simulink model "FSAC2021"  (R2014a)
settings: Solver=FixedStepDiscrete  StartTime=0.0  StopTime=inf  FixedStep=0.0005  RelTol=1e-3
model workspace (MAT data in the model file):
  MCOS : class17 (value not decoded)
  MCOS : class17 (value not decoded)
  MCOS : class17 (value not decoded)
  MCOS : class17 (value not decoded)
  MCOS : class17 (value not decoded)
  MCOS : class17 (value not decoded)
  MCOS : class17 (value not decoded)
  MCOS : class17 (value not decoded)
  MCOS : class17 (value not decoded)
  MCOS : class17 (value not decoded)
  MCOS : class17 (value not decoded)
  MCOS : class17 (value not decoded)
  MCOS : class17 (value not decoded)
  MCOS : class17 (value not decoded)
  MCOS : class17 (value not decoded)
  MCOS : class17 (value not decoded)
  MCOS : class17 (value not decoded)
  MCOS : class17 (value not decoded)
  MCOS : class17 (value not decoded)
  BUZZER_START = 1
  MCOS : class17 (value not decoded)
  MCOS : class17 (value not decoded)
  MCOS : class17 (value not decoded)
  MCOS : class17 (value not decoded)
  MCOS : class17 (value not decoded)
  MCOS : class17 (value not decoded)
  MCOS : class17 (value not decoded)
  MCOS : class17 (value not decoded)
  MCOS : class17 (value not decoded)
  MCOS : class17 (value not decoded)
  MCOS : class17 (value not decoded)
  MCOS : class17 (value not decoded)
  MCOS : class17 (value not decoded)
  MCOS : class17 (value not decoded)
  MCOS : class17 (value not decoded)
  MCOS : class17 (value not decoded)
  MCOS : class17 (value not decoded)
  MCOS : class17 (value not decoded)
  MCOS : class17 (value not decoded)
  MCOS : class17 (value not decoded)
  MCOS : class17 (value not decoded)
  MCOS : class17 (value not decoded)
  MCOS : class17 (value not decoded)
  MCOS : class17 (value not decoded)
  MCOS : class17 (value not decoded)
  MCOS : class17 (value not decoded)
  MCOS : class17 (value not decoded)
  MCOS : class17 (value not decoded)
  MCOS : class17 (value not decoded)
  MCOS : class17 (value not decoded)
  MCOS : class17 (value not decoded)
  MCOS : class17 (value not decoded)
  MCOS : class17 (value not decoded)
  MCOS : class17 (value not decoded)
  MCOS : class17 (value not decoded)
  MCOS : class17 (value not decoded)
  MCOS : class17 (value not decoded)
  MCOS : class17 (value not decoded)
  Brake = 11
  MCOS : class17 (value not decoded)
  MCOS : class17 (value not decoded)
  MCOS : class17 (value not decoded)
  MCOS : class17 (value not decoded)
  MCOS : class17 (value not decoded)
  MCOS : class17 (value not decoded)
  MCOS : class17 (value not decoded)
  MCOS : class17 (value not decoded)
  Sensor_Acc_b = 101.85
  Sensor_Acc_k = -0.0185
  Str_Sen_Orig_Angle = -341
  MCOS : class17 (value not decoded)
  Tire_D = 0.47
  T = 0.05
libraries: simulink x396, ec55xxlib x126
(part 17 of 17)

== system FSAC2021/ROUTING/TO_DCAN/Subsystem/DIAG_VEH_SENSOR/Front_wheel_angle ==
  Front_wheel_angle : Inport
  Constant{1..3,5..8} (7 alike) : Constant  Value=0  OutDataTypeStr=uint8  SampleTime=-1
  Front_wheel_angleABS : Abs
  Front_wheel_angleCS : ArithShift  BitShiftNumber=-8
  Front_wheel_angleConS : Constant  OutDataTypeStr=single
  Front_wheel_angleCosR : Constant  Value=0  OutDataTypeStr=uint8
  Front_wheel_angleROP : RelationalOperator  Operator=<  OutDataTypeStr=boolean
  Front_wheel_angleRon : Rounding  Operator=round
  Front_wheel_angleSW : Switch  Criteria=u2 ~= 0
  Front_wheel_angle_1sat : Saturate  UpperLimit=255  LowerLimit=0
  Front_wheel_angle_Convert : DataTypeConversion  OutDataTypeStr=uint8
  Front_wheel_angle_Convert1 : DataTypeConversion  OutDataTypeStr=uint32
  Front_wheel_angle_D : Product  Inputs=*/
  Front_wheel_angle_F : Constant  OutDataTypeStr=single
  Front_wheel_angle_L : simulink/Logic and Bit Operations/Bitwise Operator  logicop=AND  UseBitMask=on  BitMask=255  BitMaskRealWorld=Stored Integer
  Front_wheel_angle_O : Constant  Value=0  OutDataTypeStr=single
  Front_wheel_angle_S : ArithShift
  Front_wheel_angle_sat : Saturate  UpperLimit=127  LowerLimit=-128
  Front_wheel_angle_st : Sum  Inputs=+-
  Front_wheel_anglesubcon : Sum  Inputs=+-
  output1 : Outport
  output2 : Outport  Port=2
  output3 : Outport  Port=3
  output4 : Outport  Port=4
  output5 : Outport  Port=5
  output6 : Outport  Port=6
  output7 : Outport  Port=7
  output8 : Outport  Port=8
  wires:
  Front_wheel_angle/1 -> Front_wheel_angle_sat/1
  Front_wheel_angle_sat/1 -> Front_wheel_angle_st/1
  Front_wheel_angle_O/1 -> Front_wheel_angle_st/2
  Front_wheel_angle_st/1 -> Front_wheel_angle_D/1
  Front_wheel_angle_F/1 -> Front_wheel_angle_D/2
  Front_wheel_angle_D/1 -> Front_wheel_angleRon/1
  Front_wheel_angleRon/1 -> Front_wheel_angleROP/1, Front_wheel_angleABS/1, Front_wheel_angleSW/3
  Front_wheel_angleCosR/1 -> Front_wheel_angleROP/2
  Front_wheel_angleConS/1 -> Front_wheel_angleCS/1
  Front_wheel_angleCS/1 -> Front_wheel_anglesubcon/1
  Front_wheel_angleABS/1 -> Front_wheel_anglesubcon/2
  Front_wheel_anglesubcon/1 -> Front_wheel_angleSW/1
  Front_wheel_angleROP/1 -> Front_wheel_angleSW/2
  Front_wheel_angleSW/1 -> Front_wheel_angle_S/1
  Front_wheel_angle_S/1 -> Front_wheel_angle_1sat/1
  Front_wheel_angle_1sat/1 -> Front_wheel_angle_Convert1/1
  Front_wheel_angle_Convert1/1 -> Front_wheel_angle_L/1
  Front_wheel_angle_L/1 -> Front_wheel_angle_Convert/1
  Front_wheel_angle_Convert/1 -> output4/1
  Constant1/1 -> output1/1
  Constant2/1 -> output2/1
  Constant3/1 -> output3/1
  Constant5/1 -> output5/1
  Constant6/1 -> output6/1
  Constant7/1 -> output7/1
  Constant8/1 -> output8/1

== system FSAC2021/ROUTING/TO_DCAN/Subsystem/DIAG_VEH_SENSOR/Hydra_Prs ==
  Hydra_Prs : Inport
  Constant{1..4,6..8} (7 alike) : Constant  Value=0  OutDataTypeStr=uint8  SampleTime=-1
  Hydra_PrsRon : Rounding  Operator=round
  Hydra_Prs_1sat : Saturate  UpperLimit=255  LowerLimit=0
  Hydra_Prs_Convert : DataTypeConversion  OutDataTypeStr=uint8
  Hydra_Prs_Convert1 : DataTypeConversion  OutDataTypeStr=uint32
  Hydra_Prs_D : Product  Inputs=*/
  Hydra_Prs_F : Constant  Value=0.1  OutDataTypeStr=single
  Hydra_Prs_L : simulink/Logic and Bit Operations/Bitwise Operator  logicop=AND  UseBitMask=on  BitMask=255  BitMaskRealWorld=Stored Integer
  Hydra_Prs_O : Constant  Value=0  OutDataTypeStr=single
  Hydra_Prs_S : ArithShift
  Hydra_Prs_sat : Saturate  UpperLimit=25.5  LowerLimit=0
  Hydra_Prs_st : Sum  Inputs=+-
  output1 : Outport
  output2 : Outport  Port=2
  output3 : Outport  Port=3
  output4 : Outport  Port=4
  output5 : Outport  Port=5
  output6 : Outport  Port=6
  output7 : Outport  Port=7
  output8 : Outport  Port=8
  wires:
  Hydra_Prs/1 -> Hydra_Prs_sat/1
  Hydra_Prs_sat/1 -> Hydra_Prs_st/1
  Hydra_Prs_O/1 -> Hydra_Prs_st/2
  Hydra_Prs_st/1 -> Hydra_Prs_D/1
  Hydra_Prs_F/1 -> Hydra_Prs_D/2
  Hydra_Prs_D/1 -> Hydra_PrsRon/1
  Hydra_PrsRon/1 -> Hydra_Prs_S/1
  Hydra_Prs_S/1 -> Hydra_Prs_1sat/1
  Hydra_Prs_1sat/1 -> Hydra_Prs_Convert1/1
  Hydra_Prs_Convert1/1 -> Hydra_Prs_L/1
  Hydra_Prs_L/1 -> Hydra_Prs_Convert/1
  Hydra_Prs_Convert/1 -> output5/1
  Constant1/1 -> output1/1
  Constant2/1 -> output2/1
  Constant3/1 -> output3/1
  Constant4/1 -> output4/1
  Constant6/1 -> output6/1
  Constant7/1 -> output7/1
  Constant8/1 -> output8/1

== system FSAC2021/ROUTING/TO_DCAN/Subsystem/DIAG_VEH_SENSOR/Mtr_Input_Volt ==
  Mtr_Input_Volt : Inport
  Constant{1,3..8} (7 alike) : Constant  Value=0  OutDataTypeStr=uint8  SampleTime=-1
  Mtr_Input_VoltRon : Rounding  Operator=round
  Mtr_Input_Volt_1sat : Saturate  UpperLimit=255  LowerLimit=0
  Mtr_Input_Volt_Convert : DataTypeConversion  OutDataTypeStr=uint8
  Mtr_Input_Volt_Convert1 : DataTypeConversion  OutDataTypeStr=uint32
  Mtr_Input_Volt_D : Product  Inputs=*/
  Mtr_Input_Volt_F : Constant  OutDataTypeStr=single
  Mtr_Input_Volt_L : simulink/Logic and Bit Operations/Bitwise Operator  logicop=AND  UseBitMask=on  BitMask=255  BitMaskRealWorld=Stored Integer
  Mtr_Input_Volt_O : Constant  Value=0  OutDataTypeStr=single
  Mtr_Input_Volt_S : ArithShift
  Mtr_Input_Volt_sat : Saturate  UpperLimit=255  LowerLimit=0
  Mtr_Input_Volt_st : Sum  Inputs=+-
  output1 : Outport
  output2 : Outport  Port=2
  output3 : Outport  Port=3
  output4 : Outport  Port=4
  output5 : Outport  Port=5
  output6 : Outport  Port=6
  output7 : Outport  Port=7
  output8 : Outport  Port=8
  wires:
  Mtr_Input_Volt/1 -> Mtr_Input_Volt_sat/1
  Mtr_Input_Volt_sat/1 -> Mtr_Input_Volt_st/1
  Mtr_Input_Volt_O/1 -> Mtr_Input_Volt_st/2
  Mtr_Input_Volt_st/1 -> Mtr_Input_Volt_D/1
  Mtr_Input_Volt_F/1 -> Mtr_Input_Volt_D/2
  Mtr_Input_Volt_D/1 -> Mtr_Input_VoltRon/1
  Mtr_Input_VoltRon/1 -> Mtr_Input_Volt_S/1
  Mtr_Input_Volt_S/1 -> Mtr_Input_Volt_1sat/1
  Mtr_Input_Volt_1sat/1 -> Mtr_Input_Volt_Convert1/1
  Mtr_Input_Volt_Convert1/1 -> Mtr_Input_Volt_L/1
  Mtr_Input_Volt_L/1 -> Mtr_Input_Volt_Convert/1
  Mtr_Input_Volt_Convert/1 -> output2/1
  Constant1/1 -> output1/1
  Constant3/1 -> output3/1
  Constant4/1 -> output4/1
  Constant5/1 -> output5/1
  Constant6/1 -> output6/1
  Constant7/1 -> output7/1
  Constant8/1 -> output8/1

== system FSAC2021/ROUTING/TO_DCAN/Subsystem/DIAG_VEH_SENSOR/Pedal_Acc ==
  Pedal_Acc : Inport
  Constant{1..6} (6 alike) : Constant  Value=0  OutDataTypeStr=uint8  SampleTime=-1
  Pedal_AccBitCov : DataTypeConversion  OutDataTypeStr=uint8
  Pedal_AccCOV : DataTypeConversion  OutDataTypeStr=uint8
  Pedal_AccRon : Rounding  Operator=round
  Pedal_Acc_1sat : Saturate  UpperLimit=16256  LowerLimit=0
  Pedal_Acc_And : simulink/Logic and Bit Operations/Bitwise Operator  logicop=AND  UseBitMask=off  NumInputPorts=2  BitMask=bin2dec('11011001')  BitMaskRealWorld=Stored Integer
  Pedal_Acc_And_C : Constant  Value=255  OutDataTypeStr=uint32
  Pedal_Acc_Convert : DataTypeConversion  OutDataTypeStr=uint32
  Pedal_Acc_D : Product  Inputs=*/
  Pedal_Acc_D1 : Product  Inputs=*/
  Pedal_Acc_F : Constant  OutDataTypeStr=single
  Pedal_Acc_L : simulink/Logic and Bit Operations/Bitwise Operator  logicop=AND  UseBitMask=on  BitMask=16256  BitMaskRealWorld=Stored Integer
  Pedal_Acc_O : Constant  Value=0  OutDataTypeStr=single
  Pedal_Acc_S : ArithShift  BitShiftNumber=-7
  Pedal_Acc_sat : Saturate  UpperLimit=127  LowerLimit=0
  Pedal_Acc_st : Sum  Inputs=+-
  Pedal_Accoutput7_C : Constant  Value=256
  output1 : Outport
  output2 : Outport  Port=2
  output3 : Outport  Port=3
  output4 : Outport  Port=4
  output5 : Outport  Port=5
  output6 : Outport  Port=6
  output7 : Outport  Port=7
  output8 : Outport  Port=8
  wires:
  Pedal_Acc/1 -> Pedal_Acc_sat/1
  Pedal_Acc_sat/1 -> Pedal_Acc_st/1
  Pedal_Acc_O/1 -> Pedal_Acc_st/2
  Pedal_Acc_st/1 -> Pedal_Acc_D/1
  Pedal_Acc_F/1 -> Pedal_Acc_D/2
  Pedal_Acc_D/1 -> Pedal_AccRon/1
  Pedal_AccRon/1 -> Pedal_Acc_S/1
  Pedal_Acc_S/1 -> Pedal_Acc_1sat/1
  Pedal_Acc_1sat/1 -> Pedal_Acc_Convert/1
  Pedal_Acc_Convert/1 -> Pedal_Acc_L/1
  Pedal_Acc_L/1 -> Pedal_Acc_D1/1, Pedal_Acc_And/1
  Pedal_Accoutput7_C/1 -> Pedal_Acc_D1/2
  Pedal_Acc_D1/1 -> Pedal_AccCOV/1
  Pedal_AccCOV/1 -> output7/1
  Pedal_Acc_And_C/1 -> Pedal_Acc_And/2
  Pedal_Acc_And/1 -> Pedal_AccBitCov/1
  Pedal_AccBitCov/1 -> output8/1
  Constant1/1 -> output1/1
  Constant2/1 -> output2/1
  Constant3/1 -> output3/1
  Constant4/1 -> output4/1
  Constant5/1 -> output5/1
  Constant6/1 -> output6/1

== system FSAC2021/ROUTING/TO_DCAN/Subsystem/DIAG_VEH_SENSOR/Pedal_Brake ==
  Pedal_Brake : Inport
  Constant{1..7} (7 alike) : Constant  Value=0  OutDataTypeStr=uint8  SampleTime=-1
  Pedal_BrakeRon : Rounding  Operator=round
  Pedal_Brake_1sat : Saturate  UpperLimit=127  LowerLimit=0
  Pedal_Brake_Convert : DataTypeConversion  OutDataTypeStr=uint8
  Pedal_Brake_Convert1 : DataTypeConversion  OutDataTypeStr=uint32
  Pedal_Brake_D : Product  Inputs=*/
  Pedal_Brake_F : Constant  OutDataTypeStr=single
  Pedal_Brake_L : simulink/Logic and Bit Operations/Bitwise Operator  logicop=AND  UseBitMask=on  BitMask=127  BitMaskRealWorld=Stored Integer
  Pedal_Brake_O : Constant  Value=0  OutDataTypeStr=single
  Pedal_Brake_S : ArithShift
  Pedal_Brake_sat : Saturate  UpperLimit=127  LowerLimit=0
  Pedal_Brake_st : Sum  Inputs=+-
  output1 : Outport
  output2 : Outport  Port=2
  output3 : Outport  Port=3
  output4 : Outport  Port=4
  output5 : Outport  Port=5
  output6 : Outport  Port=6
  output7 : Outport  Port=7
  output8 : Outport  Port=8
  wires:
  Pedal_Brake/1 -> Pedal_Brake_sat/1
  Pedal_Brake_sat/1 -> Pedal_Brake_st/1
  Pedal_Brake_O/1 -> Pedal_Brake_st/2
  Pedal_Brake_st/1 -> Pedal_Brake_D/1
  Pedal_Brake_F/1 -> Pedal_Brake_D/2
  Pedal_Brake_D/1 -> Pedal_BrakeRon/1
  Pedal_BrakeRon/1 -> Pedal_Brake_S/1
  Pedal_Brake_S/1 -> Pedal_Brake_1sat/1
  Pedal_Brake_1sat/1 -> Pedal_Brake_Convert1/1
  Pedal_Brake_Convert1/1 -> Pedal_Brake_L/1
  Pedal_Brake_L/1 -> Pedal_Brake_Convert/1
  Pedal_Brake_Convert/1 -> output8/1
  Constant1/1 -> output1/1
  Constant2/1 -> output2/1
  Constant3/1 -> output3/1
  Constant4/1 -> output4/1
  Constant5/1 -> output5/1
  Constant6/1 -> output6/1
  Constant7/1 -> output7/1

== system FSAC2021/ROUTING/TO_DCAN/Subsystem/DIAG_VEH_SENSOR/Veh_Current_Speed ==
  Veh_Current_Speed : Inport
  Constant{1..5,8} (6 alike) : Constant  Value=0  OutDataTypeStr=uint8  SampleTime=-1
  Veh_Current_SpeedBitCov : DataTypeConversion  OutDataTypeStr=uint8
  Veh_Current_SpeedCOV : DataTypeConversion  OutDataTypeStr=uint8
  Veh_Current_SpeedRon : Rounding  Operator=round
  Veh_Current_Speed_1sat : Saturate  UpperLimit=65472  LowerLimit=0
  Veh_Current_Speed_And : simulink/Logic and Bit Operations/Bitwise Operator  logicop=AND  UseBitMask=off  NumInputPorts=2  BitMask=bin2dec('11011001')  BitMaskRealWorld=Stored Integer
  Veh_Current_Speed_And_C : Constant  Value=255  OutDataTypeStr=uint32
  Veh_Current_Speed_Convert : DataTypeConversion  OutDataTypeStr=uint32
  Veh_Current_Speed_D : Product  Inputs=*/
  Veh_Current_Speed_D1 : Product  Inputs=*/
  Veh_Current_Speed_F : Constant  Value=0.1  OutDataTypeStr=single
  Veh_Current_Speed_L : simulink/Logic and Bit Operations/Bitwise Operator  logicop=AND  UseBitMask=on  BitMask=65472  BitMaskRealWorld=Stored Integer
  Veh_Current_Speed_O : Constant  Value=0  OutDataTypeStr=single
  Veh_Current_Speed_S : ArithShift  BitShiftNumber=-6
  Veh_Current_Speed_sat : Saturate  UpperLimit=102.3  LowerLimit=0
  Veh_Current_Speed_st : Sum  Inputs=+-
  Veh_Current_Speedoutput6_C : Constant  Value=256
  output1 : Outport
  output2 : Outport  Port=2
  output3 : Outport  Port=3
  output4 : Outport  Port=4
  output5 : Outport  Port=5
  output6 : Outport  Port=6
  output7 : Outport  Port=7
  output8 : Outport  Port=8
  wires:
  Veh_Current_Speed/1 -> Veh_Current_Speed_sat/1
  Veh_Current_Speed_sat/1 -> Veh_Current_Speed_st/1
  Veh_Current_Speed_O/1 -> Veh_Current_Speed_st/2
  Veh_Current_Speed_st/1 -> Veh_Current_Speed_D/1
  Veh_Current_Speed_F/1 -> Veh_Current_Speed_D/2
  Veh_Current_Speed_D/1 -> Veh_Current_SpeedRon/1
  Veh_Current_SpeedRon/1 -> Veh_Current_Speed_S/1
  Veh_Current_Speed_S/1 -> Veh_Current_Speed_1sat/1
  Veh_Current_Speed_1sat/1 -> Veh_Current_Speed_Convert/1
  Veh_Current_Speed_Convert/1 -> Veh_Current_Speed_L/1
  Veh_Current_Speed_L/1 -> Veh_Current_Speed_D1/1, Veh_Current_Speed_And/1
  Veh_Current_Speedoutput6_C/1 -> Veh_Current_Speed_D1/2
  Veh_Current_Speed_D1/1 -> Veh_Current_SpeedCOV/1
  Veh_Current_SpeedCOV/1 -> output6/1
  Veh_Current_Speed_And_C/1 -> Veh_Current_Speed_And/2
  Veh_Current_Speed_And/1 -> Veh_Current_SpeedBitCov/1
  Veh_Current_SpeedBitCov/1 -> output7/1
  Constant1/1 -> output1/1
  Constant2/1 -> output2/1
  Constant3/1 -> output3/1
  Constant4/1 -> output4/1
  Constant5/1 -> output5/1
  Constant8/1 -> output8/1

== system FSAC2021/ROUTING/TO_DCAN/Subsystem/DIAG_WHL_SPD/FL_Whl_Spd ==
  FL_Whl_Spd : Inport
  Constant{3..8} (6 alike) : Constant  Value=0  OutDataTypeStr=uint8  SampleTime=-1
  FL_Whl_SpdBitCov : DataTypeConversion  OutDataTypeStr=uint8
  FL_Whl_SpdCOV : DataTypeConversion  OutDataTypeStr=uint8
  FL_Whl_SpdRon : Rounding  Operator=round
  FL_Whl_Spd_1sat : Saturate  UpperLimit=65535  LowerLimit=0
  FL_Whl_Spd_And : simulink/Logic and Bit Operations/Bitwise Operator  logicop=AND  UseBitMask=off  NumInputPorts=2  BitMask=bin2dec('11011001')  BitMaskRealWorld=Stored Integer
  FL_Whl_Spd_And_C : Constant  Value=255  OutDataTypeStr=uint32
  FL_Whl_Spd_Convert : DataTypeConversion  OutDataTypeStr=uint32
  FL_Whl_Spd_D : Product  Inputs=*/
  FL_Whl_Spd_D1 : Product  Inputs=*/
  FL_Whl_Spd_F : Constant  OutDataTypeStr=single
  FL_Whl_Spd_L : simulink/Logic and Bit Operations/Bitwise Operator  logicop=AND  UseBitMask=on  BitMask=65535  BitMaskRealWorld=Stored Integer
  FL_Whl_Spd_O : Constant  Value=0  OutDataTypeStr=single
  FL_Whl_Spd_S : ArithShift
  FL_Whl_Spd_sat : Saturate  UpperLimit=65535  LowerLimit=0
  FL_Whl_Spd_st : Sum  Inputs=+-
  FL_Whl_Spdoutput1_C : Constant  Value=256
  output1 : Outport
  output2 : Outport  Port=2
  output3 : Outport  Port=3
  output4 : Outport  Port=4
  output5 : Outport  Port=5
  output6 : Outport  Port=6
  output7 : Outport  Port=7
  output8 : Outport  Port=8
  wires:
  FL_Whl_Spd/1 -> FL_Whl_Spd_sat/1
  FL_Whl_Spd_sat/1 -> FL_Whl_Spd_st/1
  FL_Whl_Spd_O/1 -> FL_Whl_Spd_st/2
  FL_Whl_Spd_st/1 -> FL_Whl_Spd_D/1
  FL_Whl_Spd_F/1 -> FL_Whl_Spd_D/2
  FL_Whl_Spd_D/1 -> FL_Whl_SpdRon/1
  FL_Whl_SpdRon/1 -> FL_Whl_Spd_S/1
  FL_Whl_Spd_S/1 -> FL_Whl_Spd_1sat/1
  FL_Whl_Spd_1sat/1 -> FL_Whl_Spd_Convert/1
  FL_Whl_Spd_Convert/1 -> FL_Whl_Spd_L/1
  FL_Whl_Spd_L/1 -> FL_Whl_Spd_D1/1, FL_Whl_Spd_And/1
  FL_Whl_Spdoutput1_C/1 -> FL_Whl_Spd_D1/2
  FL_Whl_Spd_D1/1 -> FL_Whl_SpdCOV/1
  FL_Whl_SpdCOV/1 -> output1/1
  FL_Whl_Spd_And_C/1 -> FL_Whl_Spd_And/2
  FL_Whl_Spd_And/1 -> FL_Whl_SpdBitCov/1
  FL_Whl_SpdBitCov/1 -> output2/1
  Constant3/1 -> output3/1
  Constant4/1 -> output4/1
  Constant5/1 -> output5/1
  Constant6/1 -> output6/1
  Constant7/1 -> output7/1
  Constant8/1 -> output8/1

== system FSAC2021/ROUTING/TO_DCAN/Subsystem/DIAG_WHL_SPD/FR_Whl_Spd ==
  FR_Whl_Spd : Inport
  Constant{1..2,5..8} (6 alike) : Constant  Value=0  OutDataTypeStr=uint8  SampleTime=-1
  FR_Whl_SpdBitCov : DataTypeConversion  OutDataTypeStr=uint8
  FR_Whl_SpdCOV : DataTypeConversion  OutDataTypeStr=uint8
  FR_Whl_SpdRon : Rounding  Operator=round
  FR_Whl_Spd_1sat : Saturate  UpperLimit=65535  LowerLimit=0
  FR_Whl_Spd_And : simulink/Logic and Bit Operations/Bitwise Operator  logicop=AND  UseBitMask=off  NumInputPorts=2  BitMask=bin2dec('11011001')  BitMaskRealWorld=Stored Integer
  FR_Whl_Spd_And_C : Constant  Value=255  OutDataTypeStr=uint32
  FR_Whl_Spd_Convert : DataTypeConversion  OutDataTypeStr=uint32
  FR_Whl_Spd_D : Product  Inputs=*/
  FR_Whl_Spd_D1 : Product  Inputs=*/
  FR_Whl_Spd_F : Constant  OutDataTypeStr=single
  FR_Whl_Spd_L : simulink/Logic and Bit Operations/Bitwise Operator  logicop=AND  UseBitMask=on  BitMask=65535  BitMaskRealWorld=Stored Integer
  FR_Whl_Spd_O : Constant  Value=0  OutDataTypeStr=single
  FR_Whl_Spd_S : ArithShift
  FR_Whl_Spd_sat : Saturate  UpperLimit=65535  LowerLimit=0
  FR_Whl_Spd_st : Sum  Inputs=+-
  FR_Whl_Spdoutput3_C : Constant  Value=256
  output1 : Outport
  output2 : Outport  Port=2
  output3 : Outport  Port=3
  output4 : Outport  Port=4
  output5 : Outport  Port=5
  output6 : Outport  Port=6
  output7 : Outport  Port=7
  output8 : Outport  Port=8
  wires:
  FR_Whl_Spd/1 -> FR_Whl_Spd_sat/1
  FR_Whl_Spd_sat/1 -> FR_Whl_Spd_st/1
  FR_Whl_Spd_O/1 -> FR_Whl_Spd_st/2
  FR_Whl_Spd_st/1 -> FR_Whl_Spd_D/1
  FR_Whl_Spd_F/1 -> FR_Whl_Spd_D/2
  FR_Whl_Spd_D/1 -> FR_Whl_SpdRon/1
  FR_Whl_SpdRon/1 -> FR_Whl_Spd_S/1
  FR_Whl_Spd_S/1 -> FR_Whl_Spd_1sat/1
  FR_Whl_Spd_1sat/1 -> FR_Whl_Spd_Convert/1
  FR_Whl_Spd_Convert/1 -> FR_Whl_Spd_L/1
  FR_Whl_Spd_L/1 -> FR_Whl_Spd_D1/1, FR_Whl_Spd_And/1
  FR_Whl_Spdoutput3_C/1 -> FR_Whl_Spd_D1/2
  FR_Whl_Spd_D1/1 -> FR_Whl_SpdCOV/1
  FR_Whl_SpdCOV/1 -> output3/1
  FR_Whl_Spd_And_C/1 -> FR_Whl_Spd_And/2
  FR_Whl_Spd_And/1 -> FR_Whl_SpdBitCov/1
  FR_Whl_SpdBitCov/1 -> output4/1
  Constant1/1 -> output1/1
  Constant2/1 -> output2/1
  Constant5/1 -> output5/1
  Constant6/1 -> output6/1
  Constant7/1 -> output7/1
  Constant8/1 -> output8/1

== system FSAC2021/ROUTING/TO_DCAN/Subsystem/DIAG_WHL_SPD/RL_Whl_Spd ==
  RL_Whl_Spd : Inport
  Constant{1..4,7..8} (6 alike) : Constant  Value=0  OutDataTypeStr=uint8  SampleTime=-1
  RL_Whl_SpdBitCov : DataTypeConversion  OutDataTypeStr=uint8
  RL_Whl_SpdCOV : DataTypeConversion  OutDataTypeStr=uint8
  RL_Whl_SpdRon : Rounding  Operator=round
  RL_Whl_Spd_1sat : Saturate  UpperLimit=65535  LowerLimit=0
  RL_Whl_Spd_And : simulink/Logic and Bit Operations/Bitwise Operator  logicop=AND  UseBitMask=off  NumInputPorts=2  BitMask=bin2dec('11011001')  BitMaskRealWorld=Stored Integer
  RL_Whl_Spd_And_C : Constant  Value=255  OutDataTypeStr=uint32
  RL_Whl_Spd_Convert : DataTypeConversion  OutDataTypeStr=uint32
  RL_Whl_Spd_D : Product  Inputs=*/
  RL_Whl_Spd_D1 : Product  Inputs=*/
  RL_Whl_Spd_F : Constant  OutDataTypeStr=single
  RL_Whl_Spd_L : simulink/Logic and Bit Operations/Bitwise Operator  logicop=AND  UseBitMask=on  BitMask=65535  BitMaskRealWorld=Stored Integer
  RL_Whl_Spd_O : Constant  Value=0  OutDataTypeStr=single
  RL_Whl_Spd_S : ArithShift
  RL_Whl_Spd_sat : Saturate  UpperLimit=65535  LowerLimit=0
  RL_Whl_Spd_st : Sum  Inputs=+-
  RL_Whl_Spdoutput5_C : Constant  Value=256
  output1 : Outport
  output2 : Outport  Port=2
  output3 : Outport  Port=3
  output4 : Outport  Port=4
  output5 : Outport  Port=5
  output6 : Outport  Port=6
  output7 : Outport  Port=7
  output8 : Outport  Port=8
  wires:
  RL_Whl_Spd/1 -> RL_Whl_Spd_sat/1
  RL_Whl_Spd_sat/1 -> RL_Whl_Spd_st/1
  RL_Whl_Spd_O/1 -> RL_Whl_Spd_st/2
  RL_Whl_Spd_st/1 -> RL_Whl_Spd_D/1
  RL_Whl_Spd_F/1 -> RL_Whl_Spd_D/2
  RL_Whl_Spd_D/1 -> RL_Whl_SpdRon/1
  RL_Whl_SpdRon/1 -> RL_Whl_Spd_S/1
  RL_Whl_Spd_S/1 -> RL_Whl_Spd_1sat/1
  RL_Whl_Spd_1sat/1 -> RL_Whl_Spd_Convert/1
  RL_Whl_Spd_Convert/1 -> RL_Whl_Spd_L/1
  RL_Whl_Spd_L/1 -> RL_Whl_Spd_D1/1, RL_Whl_Spd_And/1
  RL_Whl_Spdoutput5_C/1 -> RL_Whl_Spd_D1/2
  RL_Whl_Spd_D1/1 -> RL_Whl_SpdCOV/1
  RL_Whl_SpdCOV/1 -> output5/1
  RL_Whl_Spd_And_C/1 -> RL_Whl_Spd_And/2
  RL_Whl_Spd_And/1 -> RL_Whl_SpdBitCov/1
  RL_Whl_SpdBitCov/1 -> output6/1
  Constant1/1 -> output1/1
  Constant2/1 -> output2/1
  Constant3/1 -> output3/1
  Constant4/1 -> output4/1
  Constant7/1 -> output7/1
  Constant8/1 -> output8/1

== system FSAC2021/ROUTING/TO_DCAN/Subsystem/DIAG_WHL_SPD/RR_Whl_Spd ==
  RR_Whl_Spd : Inport
  Constant{1..6} (6 alike) : Constant  Value=0  OutDataTypeStr=uint8  SampleTime=-1
  RR_Whl_SpdBitCov : DataTypeConversion  OutDataTypeStr=uint8
  RR_Whl_SpdCOV : DataTypeConversion  OutDataTypeStr=uint8
  RR_Whl_SpdRon : Rounding  Operator=round
  RR_Whl_Spd_1sat : Saturate  UpperLimit=65535  LowerLimit=0
  RR_Whl_Spd_And : simulink/Logic and Bit Operations/Bitwise Operator  logicop=AND  UseBitMask=off  NumInputPorts=2  BitMask=bin2dec('11011001')  BitMaskRealWorld=Stored Integer
  RR_Whl_Spd_And_C : Constant  Value=255  OutDataTypeStr=uint32
  RR_Whl_Spd_Convert : DataTypeConversion  OutDataTypeStr=uint32
  RR_Whl_Spd_D : Product  Inputs=*/
  RR_Whl_Spd_D1 : Product  Inputs=*/
  RR_Whl_Spd_F : Constant  OutDataTypeStr=single
  RR_Whl_Spd_L : simulink/Logic and Bit Operations/Bitwise Operator  logicop=AND  UseBitMask=on  BitMask=65535  BitMaskRealWorld=Stored Integer
  RR_Whl_Spd_O : Constant  Value=0  OutDataTypeStr=single
  RR_Whl_Spd_S : ArithShift
  RR_Whl_Spd_sat : Saturate  UpperLimit=65535  LowerLimit=0
  RR_Whl_Spd_st : Sum  Inputs=+-
  RR_Whl_Spdoutput7_C : Constant  Value=256
  output1 : Outport
  output2 : Outport  Port=2
  output3 : Outport  Port=3
  output4 : Outport  Port=4
  output5 : Outport  Port=5
  output6 : Outport  Port=6
  output7 : Outport  Port=7
  output8 : Outport  Port=8
  wires:
  RR_Whl_Spd/1 -> RR_Whl_Spd_sat/1
  RR_Whl_Spd_sat/1 -> RR_Whl_Spd_st/1
  RR_Whl_Spd_O/1 -> RR_Whl_Spd_st/2
  RR_Whl_Spd_st/1 -> RR_Whl_Spd_D/1
  RR_Whl_Spd_F/1 -> RR_Whl_Spd_D/2
  RR_Whl_Spd_D/1 -> RR_Whl_SpdRon/1
  RR_Whl_SpdRon/1 -> RR_Whl_Spd_S/1
  RR_Whl_Spd_S/1 -> RR_Whl_Spd_1sat/1
  RR_Whl_Spd_1sat/1 -> RR_Whl_Spd_Convert/1
  RR_Whl_Spd_Convert/1 -> RR_Whl_Spd_L/1
  RR_Whl_Spd_L/1 -> RR_Whl_Spd_D1/1, RR_Whl_Spd_And/1
  RR_Whl_Spdoutput7_C/1 -> RR_Whl_Spd_D1/2
  RR_Whl_Spd_D1/1 -> RR_Whl_SpdCOV/1
  RR_Whl_SpdCOV/1 -> output7/1
  RR_Whl_Spd_And_C/1 -> RR_Whl_Spd_And/2
  RR_Whl_Spd_And/1 -> RR_Whl_SpdBitCov/1
  RR_Whl_SpdBitCov/1 -> output8/1
  Constant1/1 -> output1/1
  Constant2/1 -> output2/1
  Constant3/1 -> output3/1
  Constant4/1 -> output4/1
  Constant5/1 -> output5/1
  Constant6/1 -> output6/1

== system FSAC2021/VCU_CAN_Read/PCANA(RES、AMI、MOTEC、BRAKE、STEER_SENSOR、IPC)/MOTEC_MOTION /MOTEC_MOTION/Motec_Currt_Ang_Sub ==
  In1 : Inport
  Out1 : Outport
  wires:
  In1/1 -> Out1/1

== system FSAC2021/VCU_CAN_Read/PCANA(RES、AMI、MOTEC、BRAKE、STEER_SENSOR、IPC)/MOTEC_MOTION /MOTEC_MOTION/Motec_Currt_Current_Sub ==
  In1 : Inport
  Out1 : Outport
  wires:
  In1/1 -> Out1/1

== system FSAC2021/VCU_CAN_Read/PCANA(RES、AMI、MOTEC、BRAKE、STEER_SENSOR、IPC)/MOTEC_MOTION /MOTEC_MOTION/Motec_Currt_Position_Sub ==
  In1 : Inport
  Out1 : Outport
  wires:
  In1/1 -> Out1/1

== system FSAC2021/VCU_CAN_Read/PCANA(RES、AMI、MOTEC、BRAKE、STEER_SENSOR、IPC)/Str_Emergency /MOTEC_EMERGENCY/Str_Curr_Error_Fault_Sub ==
  In1 : Inport
  Out1 : Outport
  wires:
  In1/1 -> Out1/1

== system FSAC2021/VCU_CAN_Read/PCANA(RES、AMI、MOTEC、BRAKE、STEER_SENSOR、IPC)/Str_Emergency /MOTEC_EMERGENCY/Str_Encoder_Error_Sub ==
  In1 : Inport
  Out1 : Outport
  wires:
  In1/1 -> Out1/1

== system FSAC2021/VCU_CAN_Read/PCANA(RES、AMI、MOTEC、BRAKE、STEER_SENSOR、IPC)/Str_Emergency /MOTEC_EMERGENCY/Str_Flash_Error_Sub ==
  In1 : Inport
  Out1 : Outport
  wires:
  In1/1 -> Out1/1

== system FSAC2021/VCU_CAN_Read/PCANA(RES、AMI、MOTEC、BRAKE、STEER_SENSOR、IPC)/Str_Emergency /MOTEC_EMERGENCY/Str_I2t_Alarm_Sub ==
  In1 : Inport
  Out1 : Outport
  wires:
  In1/1 -> Out1/1

== system FSAC2021/VCU_CAN_Read/PCANA(RES、AMI、MOTEC、BRAKE、STEER_SENSOR、IPC)/Str_Emergency /MOTEC_EMERGENCY/Str_I2t_Warning_Sub ==
  In1 : Inport
  Out1 : Outport
  wires:
  In1/1 -> Out1/1

== system FSAC2021/VCU_CAN_Read/PCANA(RES、AMI、MOTEC、BRAKE、STEER_SENSOR、IPC)/Str_Emergency /MOTEC_EMERGENCY/Str_Limit_Pos_Alarm_Sub ==
  In1 : Inport
  Out1 : Outport
  wires:
  In1/1 -> Out1/1

== system FSAC2021/VCU_CAN_Read/PCANA(RES、AMI、MOTEC、BRAKE、STEER_SENSOR、IPC)/Str_Emergency /MOTEC_EMERGENCY/Str_Over_PosError_Sub ==
  In1 : Inport
  Out1 : Outport
  wires:
  In1/1 -> Out1/1

== system FSAC2021/VCU_CAN_Read/PCANA(RES、AMI、MOTEC、BRAKE、STEER_SENSOR、IPC)/Str_Emergency /MOTEC_EMERGENCY/Str_Over_SpdError_Sub ==
  In1 : Inport
  Out1 : Outport
  wires:
  In1/1 -> Out1/1

== system FSAC2021/VCU_CAN_Read/PCANA(RES、AMI、MOTEC、BRAKE、STEER_SENSOR、IPC)/Str_Emergency /MOTEC_EMERGENCY/Str_Over_TopCurr_Sub ==
  In1 : Inport
  Out1 : Outport
  wires:
  In1/1 -> Out1/1

== system FSAC2021/VCU_CAN_Read/PCANA(RES、AMI、MOTEC、BRAKE、STEER_SENSOR、IPC)/Str_Emergency /MOTEC_EMERGENCY/Str_Overvolt_Warning_Sub ==
  In1 : Inport
  Out1 : Outport
  wires:
  In1/1 -> Out1/1

== system FSAC2021/VCU_CAN_Read/PCANA(RES、AMI、MOTEC、BRAKE、STEER_SENSOR、IPC)/Str_Emergency /MOTEC_EMERGENCY/Str_Para_Error_Sub ==
  In1 : Inport
  Out1 : Outport
  wires:
  In1/1 -> Out1/1

== system FSAC2021/VCU_CAN_Read/PCANA(RES、AMI、MOTEC、BRAKE、STEER_SENSOR、IPC)/Str_Emergency /MOTEC_EMERGENCY/Str_PwrMod_TempHigh_Alarm_Sub ==
  In1 : Inport
  Out1 : Outport
  wires:
  In1/1 -> Out1/1

== system FSAC2021/VCU_CAN_Read/PCANA(RES、AMI、MOTEC、BRAKE、STEER_SENSOR、IPC)/Str_Emergency /MOTEC_EMERGENCY/Str_PwrMod_TempHigh_Warning_Sub ==
  In1 : Inport
  Out1 : Outport
  wires:
  In1/1 -> Out1/1

== system FSAC2021/VCU_CAN_Read/PCANA(RES、AMI、MOTEC、BRAKE、STEER_SENSOR、IPC)/Str_Emergency /MOTEC_EMERGENCY/Str_Spd_Over_Alam_Sub ==
  In1 : Inport
  Out1 : Outport
  wires:
  In1/1 -> Out1/1

== system FSAC2021/VCU_CAN_Read/PCANA(RES、AMI、MOTEC、BRAKE、STEER_SENSOR、IPC)/Str_Emergency /MOTEC_EMERGENCY/Str_System_Error_Sub ==
  In1 : Inport
  Out1 : Outport
  wires:
  In1/1 -> Out1/1

== system FSAC2021/VCU_CAN_Read/PCANA(RES、AMI、MOTEC、BRAKE、STEER_SENSOR、IPC)/Str_Emergency /MOTEC_EMERGENCY/Str_UnderVolt_Warning_Sub ==
  In1 : Inport
  Out1 : Outport
  wires:
  In1/1 -> Out1/1

== system FSAC2021/VCU_CAN_Read/PCANB(BMS、DRIVE_MOTOR)/BMS_ALARM /BMS_HCU_ALARM/ALM_AUX_FAIL_Sub ==
  In1 : Inport
  Out1 : Outport
  wires:
  In1/1 -> Out1/1

== system FSAC2021/VCU_CAN_Read/PCANB(BMS、DRIVE_MOTOR)/BMS_ALARM /BMS_HCU_ALARM/ALM_BATT_DT_Sub ==
  In1 : Inport
  Out1 : Outport
  wires:
  In1/1 -> Out1/1

== system FSAC2021/VCU_CAN_Read/PCANB(BMS、DRIVE_MOTOR)/BMS_ALARM /BMS_HCU_ALARM/ALM_BATT_DV_Sub ==
  In1 : Inport
  Out1 : Outport
  wires:
  In1/1 -> Out1/1

== system FSAC2021/VCU_CAN_Read/PCANB(BMS、DRIVE_MOTOR)/BMS_ALARM /BMS_HCU_ALARM/ALM_BATT_OC_Sub ==
  In1 : Inport
  Out1 : Outport
  wires:
  In1/1 -> Out1/1

== system FSAC2021/VCU_CAN_Read/PCANB(BMS、DRIVE_MOTOR)/BMS_ALARM /BMS_HCU_ALARM/ALM_BATT_OV_Sub ==
  In1 : Inport
  Out1 : Outport
  wires:
  In1/1 -> Out1/1

== system FSAC2021/VCU_CAN_Read/PCANB(BMS、DRIVE_MOTOR)/BMS_ALARM /BMS_HCU_ALARM/ALM_BATT_UC_Sub ==
  In1 : Inport
  Out1 : Outport
  wires:
  In1/1 -> Out1/1

== system FSAC2021/VCU_CAN_Read/PCANB(BMS、DRIVE_MOTOR)/BMS_ALARM /BMS_HCU_ALARM/ALM_BATT_UV_Sub ==
  In1 : Inport
  Out1 : Outport
  wires:
  In1/1 -> Out1/1

== system FSAC2021/VCU_CAN_Read/PCANB(BMS、DRIVE_MOTOR)/BMS_ALARM /BMS_HCU_ALARM/ALM_BMU_FAIL_Sub ==
  In1 : Inport
  Out1 : Outport
  wires:
  In1/1 -> Out1/1

== system FSAC2021/VCU_CAN_Read/PCANB(BMS、DRIVE_MOTOR)/BMS_ALARM /BMS_HCU_ALARM/ALM_BSU_FAULT_Sub ==
  In1 : Inport
  Out1 : Outport
  wires:
  In1/1 -> Out1/1

== system FSAC2021/VCU_CAN_Read/PCANB(BMS、DRIVE_MOTOR)/BMS_ALARM /BMS_HCU_ALARM/ALM_BSU_OFFLINE_Sub ==
  In1 : Inport
  Out1 : Outport
  wires:
  In1/1 -> Out1/1

== system FSAC2021/VCU_CAN_Read/PCANB(BMS、DRIVE_MOTOR)/BMS_ALARM /BMS_HCU_ALARM/ALM_CELL_IBK_Sub ==
  In1 : Inport
  Out1 : Outport
  wires:
  In1/1 -> Out1/1

== system FSAC2021/VCU_CAN_Read/PCANB(BMS、DRIVE_MOTOR)/BMS_ALARM /BMS_HCU_ALARM/ALM_CELL_OT_Sub ==
  In1 : Inport
  Out1 : Outport
  wires:
  In1/1 -> Out1/1

== system FSAC2021/VCU_CAN_Read/PCANB(BMS、DRIVE_MOTOR)/BMS_ALARM /BMS_HCU_ALARM/ALM_CELL_OV_Sub ==
  In1 : Inport
  Out1 : Outport
  wires:
  In1/1 -> Out1/1

== system FSAC2021/VCU_CAN_Read/PCANB(BMS、DRIVE_MOTOR)/BMS_ALARM /BMS_HCU_ALARM/ALM_CELL_TBK_Sub ==
  In1 : Inport
  Out1 : Outport
  wires:
  In1/1 -> Out1/1

== system FSAC2021/VCU_CAN_Read/PCANB(BMS、DRIVE_MOTOR)/BMS_ALARM /BMS_HCU_ALARM/ALM_CELL_UT_Sub ==
  In1 : Inport
  Out1 : Outport
  wires:
  In1/1 -> Out1/1

== system FSAC2021/VCU_CAN_Read/PCANB(BMS、DRIVE_MOTOR)/BMS_ALARM /BMS_HCU_ALARM/ALM_CELL_UV_Sub ==
  In1 : Inport
  Out1 : Outport
  wires:
  In1/1 -> Out1/1

== system FSAC2021/VCU_CAN_Read/PCANB(BMS、DRIVE_MOTOR)/BMS_ALARM /BMS_HCU_ALARM/ALM_CHRG_OCS_Sub ==
  In1 : Inport
  Out1 : Outport
  wires:
  In1/1 -> Out1/1

== system FSAC2021/VCU_CAN_Read/PCANB(BMS、DRIVE_MOTOR)/BMS_ALARM /BMS_HCU_ALARM/ALM_CHRG_OCT_Sub ==
  In1 : Inport
  Out1 : Outport
  wires:
  In1/1 -> Out1/1

== system FSAC2021/VCU_CAN_Read/PCANB(BMS、DRIVE_MOTOR)/BMS_ALARM /BMS_HCU_ALARM/ALM_DSCH_OCS_Sub ==
  In1 : Inport
  Out1 : Outport
  wires:
  In1/1 -> Out1/1

== system FSAC2021/VCU_CAN_Read/PCANB(BMS、DRIVE_MOTOR)/BMS_ALARM /BMS_HCU_ALARM/ALM_DSCH_OCT_Sub ==
  In1 : Inport
  Out1 : Outport
  wires:
  In1/1 -> Out1/1

== system FSAC2021/VCU_CAN_Read/PCANB(BMS、DRIVE_MOTOR)/BMS_ALARM /BMS_HCU_ALARM/ALM_HALL_BREAK_Sub ==
  In1 : Inport
  Out1 : Outport
  wires:
  In1/1 -> Out1/1

== system FSAC2021/VCU_CAN_Read/PCANB(BMS、DRIVE_MOTOR)/BMS_ALARM /BMS_HCU_ALARM/ALM_HVREL_FAIL_Sub ==
  In1 : Inport
  Out1 : Outport
  wires:
  In1/1 -> Out1/1

== system FSAC2021/VCU_CAN_Read/PCANB(BMS、DRIVE_MOTOR)/BMS_ALARM /BMS_HCU_ALARM/ALM_LEAK_OC_Sub ==
  In1 : Inport
  Out1 : Outport
  wires:
  In1/1 -> Out1/1

== system FSAC2021/VCU_CAN_Read/PCANB(BMS、DRIVE_MOTOR)/BMS_ALARM /BMS_HCU_ALARM/ALM_PRECHRG_FAIL_Sub ==
  In1 : Inport
  Out1 : Outport
  wires:
  In1/1 -> Out1/1

== system FSAC2021/VCU_CAN_Read/PCANB(BMS、DRIVE_MOTOR)/BMS_ALARM /BMS_HCU_ALARM/ALM_VCU_OFFLINE_Sub ==
  In1 : Inport
  Out1 : Outport
  wires:
  In1/1 -> Out1/1

== system FSAC2021/VCU_CAN_Read/PCANB(BMS、DRIVE_MOTOR)/BMS_HCU_MAXV /BMS_HCU_MAXV/MaxCellVoltNo_Sub ==
  In1 : Inport
  Out1 : Outport
  wires:
  In1/1 -> Out1/1

== system FSAC2021/VCU_CAN_Read/PCANB(BMS、DRIVE_MOTOR)/BMS_HCU_MAXV /BMS_HCU_MAXV/MaxCellVolt_Sub ==
  In1 : Inport
  Out1 : Outport
  wires:
  In1/1 -> Out1/1

== system FSAC2021/VCU_CAN_Read/PCANB(BMS、DRIVE_MOTOR)/BMS_HCU_MAXV /BMS_HCU_MAXV/MinCellVoltNo_Sub ==
  In1 : Inport
  Out1 : Outport
  wires:
  In1/1 -> Out1/1

== system FSAC2021/VCU_CAN_Read/PCANB(BMS、DRIVE_MOTOR)/BMS_HCU_MAXV /BMS_HCU_MAXV/MinCellVolt_Sub ==
  In1 : Inport
  Out1 : Outport
  wires:
  In1/1 -> Out1/1

== system FSAC2021/VCU_CAN_Read/PCANB(BMS、DRIVE_MOTOR)/BMS_HCU_POWER /BMS_HCU_POWER/MaxChrCurtLimit_Sub ==
  In1 : Inport
  Out1 : Outport
  wires:
  In1/1 -> Out1/1

== system FSAC2021/VCU_CAN_Read/PCANB(BMS、DRIVE_MOTOR)/BMS_HCU_POWER /BMS_HCU_POWER/MaxChrPowerLimit_Sub ==
  In1 : Inport
  Out1 : Outport
  wires:
  In1/1 -> Out1/1

== system FSAC2021/VCU_CAN_Read/PCANB(BMS、DRIVE_MOTOR)/BMS_HCU_POWER /BMS_HCU_POWER/MaxDisCurtLimit_Sub ==
  In1 : Inport
  Out1 : Outport
  wires:
  In1/1 -> Out1/1

== system FSAC2021/VCU_CAN_Read/PCANB(BMS、DRIVE_MOTOR)/BMS_HCU_POWER /BMS_HCU_POWER/MaxDisPowerLimit_Sub ==
  In1 : Inport
  Out1 : Outport
  wires:
  In1/1 -> Out1/1

== system FSAC2021/VCU_CAN_Read/PCANB(BMS、DRIVE_MOTOR)/BMS_RELAY /BMS_HCU_RELAY/ChrCommunication_Sub ==
  In1 : Inport
  Out1 : Outport
  wires:
  In1/1 -> Out1/1

== system FSAC2021/VCU_CAN_Read/PCANB(BMS、DRIVE_MOTOR)/BMS_RELAY /BMS_HCU_RELAY/ChrReqCurr_Sub ==
  In1 : Inport
  Out1 : Outport
  wires:
  In1/1 -> Out1/1

== system FSAC2021/VCU_CAN_Read/PCANB(BMS、DRIVE_MOTOR)/BMS_RELAY /BMS_HCU_RELAY/ChrReqVolt_Sub ==
  In1 : Inport
  Out1 : Outport
  wires:
  In1/1 -> Out1/1

== system FSAC2021/VCU_CAN_Read/PCANB(BMS、DRIVE_MOTOR)/BMS_RELAY /BMS_HCU_RELAY/ChrState_Sub ==
  In1 : Inport
  Out1 : Outport
  wires:
  In1/1 -> Out1/1

== system FSAC2021/VCU_CAN_Read/PCANB(BMS、DRIVE_MOTOR)/BMS_RELAY /BMS_HCU_RELAY/NegRlyStr_Sub ==
  In1 : Inport
  Out1 : Outport
  wires:
  In1/1 -> Out1/1

== system FSAC2021/VCU_CAN_Read/PCANB(BMS、DRIVE_MOTOR)/BMS_RELAY /BMS_HCU_RELAY/OnChrRlyStr_Sub ==
  In1 : Inport
  Out1 : Outport
  wires:
  In1/1 -> Out1/1

== system FSAC2021/VCU_CAN_Read/PCANB(BMS、DRIVE_MOTOR)/BMS_RELAY /BMS_HCU_RELAY/PosRlyStr_Sub ==
  In1 : Inport
  Out1 : Outport
  wires:
  In1/1 -> Out1/1

== system FSAC2021/VCU_CAN_Read/PCANB(BMS、DRIVE_MOTOR)/BMS_RELAY /BMS_HCU_RELAY/PreRlyStr_Sub ==
  In1 : Inport
  Out1 : Outport
  wires:
  In1/1 -> Out1/1

== system FSAC2021/VCU_CAN_Read/PCANB(BMS、DRIVE_MOTOR)/BMS_RELAY /BMS_HCU_RELAY/chrOFFCC2_Sub ==
  In1 : Inport
  Out1 : Outport
  wires:
  In1/1 -> Out1/1

== system FSAC2021/VCU_CAN_Read/PCANB(BMS、DRIVE_MOTOR)/BMS_RELAY /BMS_HCU_RELAY/chrONCC_Sub ==
  In1 : Inport
  Out1 : Outport
  wires:
  In1/1 -> Out1/1

== system FSAC2021/VCU_CAN_Read/PCANB(BMS、DRIVE_MOTOR)/BMS_RELAY /BMS_HCU_RELAY/offChrRlyStr_Sub ==
  In1 : Inport
  Out1 : Outport
  wires:
  In1/1 -> Out1/1

== system FSAC2021/VCU_CAN_Read/Subsystem/BMS_HCU_INFO /BMS_HCU_INFO/BatAlmLv_Sub ==
  In1 : Inport
  Out1 : Outport
  wires:
  In1/1 -> Out1/1

== system FSAC2021/VCU_CAN_Read/Subsystem/BMS_HCU_INFO /BMS_HCU_INFO/BatCurrent_Sub ==
  In1 : Inport
  Out1 : Outport
  wires:
  In1/1 -> Out1/1

== system FSAC2021/VCU_CAN_Read/Subsystem/BMS_HCU_INFO /BMS_HCU_INFO/BatLife_Sub ==
  In1 : Inport
  Out1 : Outport
  wires:
  In1/1 -> Out1/1

== system FSAC2021/VCU_CAN_Read/Subsystem/BMS_HCU_INFO /BMS_HCU_INFO/BatSoc_Sub ==
  In1 : Inport
  Out1 : Outport
  wires:
  In1/1 -> Out1/1

== system FSAC2021/VCU_CAN_Read/Subsystem/BMS_HCU_INFO /BMS_HCU_INFO/BatSoh_Sub ==
  In1 : Inport
  Out1 : Outport
  wires:
  In1/1 -> Out1/1

== system FSAC2021/VCU_CAN_Read/Subsystem/BMS_HCU_INFO /BMS_HCU_INFO/BatState_Sub ==
  In1 : Inport
  Out1 : Outport
  wires:
  In1/1 -> Out1/1

== system FSAC2021/VCU_CAN_Read/Subsystem/BMS_HCU_INFO /BMS_HCU_INFO/BatVoltage_Sub ==
  In1 : Inport
  Out1 : Outport
  wires:
  In1/1 -> Out1/1

== system FSAC2021/VCU_CAN_Read/Subsystem1/HEARTBEAT /MOTEC_HEARTBEAT/Heartbeat_info_Sub ==
  In1 : Inport
  Out1 : Outport
  wires:
  In1/1 -> Out1/1

== system FSAC2021/VCU_CAN_Read/Subsystem2/MOTEC_STATUS /MOTEC_STATUS/Fault_Sub ==
  In1 : Inport
  Out1 : Outport
  wires:
  In1/1 -> Out1/1

== system FSAC2021/VCU_CAN_Read/Subsystem2/MOTEC_STATUS /MOTEC_STATUS/Operation_Enabled_Sub ==
  In1 : Inport
  Out1 : Outport
  wires:
  In1/1 -> Out1/1

== system FSAC2021/VCU_CAN_Read/Subsystem2/MOTEC_STATUS /MOTEC_STATUS/Quick_Stop_Sub ==
  In1 : Inport
  Out1 : Outport
  wires:
  In1/1 -> Out1/1

== system FSAC2021/VCU_CAN_Read/Subsystem2/MOTEC_STATUS /MOTEC_STATUS/Ready_Switch_On_Sub ==
  In1 : Inport
  Out1 : Outport
  wires:
  In1/1 -> Out1/1

== system FSAC2021/VCU_CAN_Read/Subsystem2/MOTEC_STATUS /MOTEC_STATUS/Switch_On_Disabled_Sub ==
  In1 : Inport
  Out1 : Outport
  wires:
  In1/1 -> Out1/1

== system FSAC2021/VCU_CAN_Read/Subsystem2/MOTEC_STATUS /MOTEC_STATUS/Swtiched_On_Sub ==
  In1 : Inport
  Out1 : Outport
  wires:
  In1/1 -> Out1/1

== system FSAC2021/VCU_CAN_Read/Subsystem2/MOTEC_STATUS /MOTEC_STATUS/Target_Reached_Sub ==
  In1 : Inport
  Out1 : Outport
  wires:
  In1/1 -> Out1/1

== system FSAC2021/VCU_CAN_Read/Subsystem2/MOTEC_STATUS /MOTEC_STATUS/Voltage_Enabled_Sub ==
  In1 : Inport
  Out1 : Outport
  wires:
  In1/1 -> Out1/1

== system FSAC2021/VCU_CAN_Read/Subsystem2/MOTEC_STATUS /MOTEC_STATUS/Warning_Sub ==
  In1 : Inport
  Out1 : Outport
  wires:
  In1/1 -> Out1/1

== stateflow chart FSAC2021/Controller/50ms_Duty/Visuality Check/Chart ==
  state Visuality_On
    en:Visual_Lights =uint8(1);
    Visual_Flag = uint8(1);
  state Visuality_Off
    en:Visual_Lights =uint8(0);
    Visual_Flag = uint8(0);
  (default) -> Visuality_On
  Visuality_On -> Visuality_Off : [after(2,sec)]
  data: Visual_Lights output uint8 size=3; Visual_Flag output uint8

== stateflow chart FSAC2021/Controller/50ms_Duty/AS_Machine ==
  state AS_Driving
    en:R2D = ON;
    ASSI_State = AS_DRIVING;
    Yellow_Light = BLINK;
    Blue_Light = OFF;
    Buzzer = BUZZER_START;
  state AS_Off
    en:ASSI_State =AS_OFF;
    System_48V_Relay = DISABLE;
    Blue_Light = OFF;
    Yellow_Light = OFF;
    VCU_Valve = ON;
    du:Manual_R2D_Detect;
    Visuality_Check;
  state AS_Ready
    en:ASSI_State = AS_READY;
    System_48V_Relay = ENABLE;
    Yellow_Light = ON;
    Blue_Light = OFF;
  state Manual_Driving
    en:
    R2D = ON;
    ASSI_State = MANUAL_DRIVING;
  state AS_Emergency
    en:
    ASSI_State = AS_EMERGENCY;
    R2D = OFF;
    Yellow_Light = OFF;
    Blue_Light = BLINK;
    Buzzer = BUZZER_EBS;
  state AS_Finished
    en:
    ASSI_State =AS_FINISH;
    R2D = OFF;
    Safety_Circuit_Relay = ON;
    System_48V_Relay = OFF;
    Blue_Light = ON;
    Yellow_Light = OFF;
  (default) -> AS_Off
  AS_Off -> AS_Ready [order 2] : [LVMS&&ASMS && TS_Flag &&...
      | AMI_State&&...
      | EBS_Flag==EBS_ARMED&&...
      | Res_Origin_Flag]
  AS_Ready -> AS_Driving [order 1] : [after(5,sec) && Res_GO]
  AS_Driving -> (junction 69) [order 2] : [EBS_Flag==EBS_ENABLE]
  (junction 69) -> AS_Emergency
  AS_Ready -> AS_Off [order 2] : [!ASMS ]
  AS_Driving -> AS_Finished [order 1] : [Veh_Spd <= 1 &&...
      | Misson_Finished ]
  AS_Ready -> AS_Emergency [order 3] : [EBS_Flag==EBS_ENABLE]
  AS_Off -> Manual_Driving [order 1] : [AMI_State == MANUAL_MODE&&...
      | TS_Flag&&...
      | !ASMS&&START_Flag]
  Manual_Driving -> AS_Off : [ !TS_Flag]
  AS_Emergency -> AS_Off : [!ASMS &&Buzzer_Overflag&&...
      |  EBS_Flag ==EBS_DISABLE]
  AS_Finished -> AS_Emergency [order 1] : [ Res_EBS]
  AS_Finished -> (junction 64) [order 2]
  (junction 65) -> AS_Off
  (junction 64) -> (junction 65) : [!ASMS  ]
  data: Blue_Light output uint8; Yellow_Light output uint8; Buzzer output uint8; TS_Flag input uint8; EBS_Flag input uint8; Safety_Circuit_Relay output uint8; System_48V_Relay output uint8; ASSI_State output uint8; Veh_Spd input single; ASMS input uint8; ON parameter uint8; OFF parameter uint8; ENABLE parameter uint8; DISABLE parameter uint8; AS_OFF parameter uint8; AS_READY parameter uint8; AS_DRIVING parameter uint8; AS_FINISH parameter uint8; AS_EMERGENCY parameter uint8; BLINK parameter uint8; EBS_DISABLE parameter uint8; EBS_ARMED parameter uint8; EBS_ENABLE parameter uint8; VCU_Valve output uint8; R2D output uint8; MANUAL_DRIVING parameter uint8; MANUAL_MODE parameter uint8; LVMS input uint8; AMI_State input uint8; Res_EBS input uint8; Res_GO input uint8; START_Flag input uint8; Misson_Finished input uint8; Buzzer_Overflag input uint8; BUZZER_START parameter uint8; BUZZER_EBS parameter uint8; TRACKDRIVE parameter uint8; Res_Origin_Flag input uint8
  events: Manual_R2D_Detect output FUNCTION_CALL_EVENT; Visuality_Check output FUNCTION_CALL_EVENT

== stateflow chart FSAC2021/DIAG/DIAG/CAN_NODE_LOSTCOM/B_M_S_Check/Chart ==
  state Normal
    en:
    Output = uint8(1);
  state Off
  state ON
  state On
    en:
    Output = uint8(0);
  (default) -> Normal
  Normal -> ON : [Input == 0&&after(500,msec)]
  ON -> Off [order 1] : [Input == uint8(1)]
  Off -> ON : [Input == uint8(0)]
  ON -> On [order 2] : after(2,sec)
  data: Input input; Output output

== stateflow chart FSAC2021/Controller/50ms_Duty/Subsystem/Chart ==
  state Task
    du:
    MODE = 3;%%车检任务
  state init
  state Manul
    du:
    MODE = 1;%手动模式
  state Driverless
    du:
    MODE = 2;%%无人驾驶模式
  (junction 15) -> Task
  init -> (junction 15) [order 3] : [AMI_Duty == 4 ]
  init -> Manul [order 1] : [AMI_Duty == 6]
  (default) -> init
  init -> Driverless [order 2] : [AMI_Duty == 1 || AMI_Duty == 2 || AMI_Duty == 3 || AMI_Duty == 5]
  Manul -> (junction 6)
  (junction 6) -> Driverless : [AMI_Duty == 1 || AMI_Duty == 2 || AMI_Duty == 3 || AMI_Duty == 5]
  data: AMI_Duty input; MODE output

== stateflow chart FSAC2021/DIAG/DIAG/CAN_NODE_LOSTCOM/B_M_S_Check/Chart1 ==
  state Normal
    en:
    Output = uint8(1);
  state Off
  state ON
  state On
    en:
    Output = uint8(0);
  (default) -> Normal
  Normal -> ON : [Input == 0]
  ON -> Off [order 1] : [Input == uint8(1)]
  Off -> ON : [Input == uint8(0)]
  ON -> On [order 2] : after(2,sec)
  data: Input input; Output output

== stateflow chart FSAC2021/Controller/200ms_Duty/Light_Subsystem2/Start_Horn/Chart ==
  state Start_Horn_ON
    en: Buzzer_Pin = ON;
  state Start_Horn_OFF
    en: Buzzer_Pin = OFF;
  (default) -> Start_Horn_ON
  Start_Horn_ON -> Start_Horn_OFF : [after(2,sec)]
  data: Buzzer_Pin output uint8; OFF parameter; ON parameter

== stateflow chart FSAC2021/Controller/200ms_Duty/Light_Subsystem2/EBS_Horn/Chart ==
  state Horn
    state EBS_Horn_ON
      en: Buzzer_Pin = ON;
    state EBS_Horn_ON1
      en:Buzzer_Pin = OFF;
    (default) -> EBS_Horn_ON
    EBS_Horn_ON1 -> EBS_Horn_ON : [after(100,msec)]
    EBS_Horn_ON -> EBS_Horn_ON1 : [after(100,msec)]
  state EBS_Horn_OFF
    en: Buzzer_Pin = OFF;
    Buzzer_Overflag = ENABLE
  (default) -> Horn
  Horn -> EBS_Horn_OFF : [after(9,sec)]
  data: Buzzer_Pin output uint8; OFF parameter; ON parameter; Buzzer_Overflag output uint8; ENABLE parameter

== stateflow chart FSAC2021/Controller/50ms_Duty/Subsystem/Subsystem2/Chart ==
  state init
    en:
    SteerCmd = 0;
    ACC = 200;
  state IN
    en:
    state Second
      du:
      SteerCmd = SteerCmd - 5;
    state Move
      du:
      SteerCmd = SteerCmd + 5;
    Move -> Second : [SteerCmd>=110]
    (default) -> Move
    Second -> Move : [SteerCmd <= -110]
  state end
    en:
    ACC = 0;
    SteerCmd = 0;
    Mission_Flag = uint8(1);
  (default) -> init
  init -> IN
  IN -> end : [after(27,sec)]
  data: Mission_Flag output; SteerCmd output; ACC output

== stateflow chart FSAC2021/DIAG/DIAG/CAN_NODE_LOSTCOM/Subsystem1/Chart2 ==
  state Normal
    en:
    Output = uint8(1);
  state Off
  state ON
  state On
    en:
    Output = uint8(0);
  (default) -> Normal
  Normal -> ON : [Input == 0]
  ON -> Off [order 1] : [Input == uint8(1)]
  Off -> ON : [Input == uint8(0)]
  ON -> On [order 2] : after(2,sec)
  data: Input input; Output output

== stateflow chart FSAC2021/DIAG/DIAG/CAN_NODE_LOSTCOM/Subsystem/Chart4 ==
  state Normal
    en:
    Output = uint8(1);
  state Off
  state ON
  state On
    en:
    Output = uint8(0);
  (default) -> Normal
  Normal -> ON : [Input == 0]
  ON -> Off [order 1] : [Input == uint8(1)]
  Off -> ON : [Input == uint8(0)]
  ON -> On [order 2] : after(2,sec)
  data: Input input; Output output

== matlab function FSAC2021/DIAG/DIAG/EBS_Diag/Truth Table ==
  settings: updateMethod=DISCRETE
  data: ASSI_State input uint8; EBS_Failure_Flag output uint8; EBS_GAS_Prs_1_Val input uint16; EBS_GAS_Prs_2_Val input uint16
function EBS_Failure_Flag = fcn(ASSI_State, EBS_GAS_Prs_1_Val, EBS_GAS_Prs_2_Val)

aVarTruthTableCondition_1 = false;
aVarTruthTableCondition_2 = false;
aVarTruthTableCondition_3 = false;
aVarTruthTableCondition_4 = false;
aVarTruthTableCondition_5 = false;


% Ready or Driving

aVarTruthTableCondition_1 = logical(ASSI_State ==2||ASSI_State ==3);


aVarTruthTableCondition_2 = logical(EBS_GAS_Prs_1_Val<0.4);


aVarTruthTableCondition_3 = logical(EBS_GAS_Prs_1_Val>=0.4);


aVarTruthTableCondition_4 = logical(EBS_GAS_Prs_2_Val<=0.4);


aVarTruthTableCondition_5 = logical(EBS_GAS_Prs_2_Val>0.4);

if (aVarTruthTableCondition_1 && aVarTruthTableCondition_2 && aVarTruthTableCondition_4)
    A1();
elseif (aVarTruthTableCondition_1 && aVarTruthTableCondition_3 && aVarTruthTableCondition_4)
    A2();
elseif (aVarTruthTableCondition_1 && aVarTruthTableCondition_3 && aVarTruthTableCondition_5)
    A1();
else % Default
    A2();
end

function A1()

% EBS_Failure

EBS_Failure_Flag=uint8(1);

function A2()

% EBS_Normal

EBS_Failure_Flag=uint8(0);

== stateflow chart FSAC2021/Controller/SteerCtr/Chart ==
  state Pre_Operation_Mode
    en:
    NMT_nodeorder = uint8(1); //开启远程节点。
    NMT_nodectrl = uint8(0);//连接所有节点。
    du:TmtNMTCAN;
  state Init
  state Move
    state Goto
      du:TmtRPDO1CAN;
      Fault_Resrt = uint8(0);
      Enable_Operation_Ctrl = uint8(1);//允许操作。
      state Origin_Pos_Set
        en:
        Position_set = (Origin_Back_Angle);//电机回位角度赋值。
        New_Set_Point_Ctrl = uint8(0);
      state Origin_Aciton_Move
        en:
        New_Set_Point_Ctrl = uint8(1);//设置新位置点。
        Abs_or_Rel_Ctrl = uint8(0);//相对位置移动。
      (default) -> Origin_Pos_Set
      Origin_Aciton_Move -> Origin_Pos_Set [order 2]
      Origin_Pos_Set -> Origin_Aciton_Move
    state Motor_Enable
      du:TmtRPDO1CAN;
      state First
        en:
        Switch_On_Ctrl = uint8(0); //
        Enable_Voltage_Ctrl = uint8(1);//允许通电。
        Quick_Stop_Ctrl = uint8(1);//禁用快速停止。
      state Second
        en:Switch_On_Ctrl = uint8(1);// 伺服使能
      (default) -> First
      First -> Second
    state Motor_Move
      du:TmtRPDO1CAN;
      enflag = uint8(1);
      state Move_Position_Set
        en:
        Enable_Operation_Ctrl = uint8(1);//允许操作。
        Position_set = int16(Steer_Go_Angle);//期望电机角度赋值
        New_Set_Point_Ctrl = uint8(0);
        Abs_or_Rel_Ctrl = uint8(0);//相对位置移动。
      state Aciton_Move
        en:
        New_Set_Point_Ctrl = uint8(1);//设置新位置点。
        Abs_or_Rel_Ctrl = uint8(1);//绝对位置移动。
      (default) -> Move_Position_Set
      Move_Position_Set -> Aciton_Move
      Aciton_Move -> Move_Position_Set
    state Wait
    state Motor_Stanby
      du:TmtSDOCAN;
      Original_Flag = uint8(1);
      state Encoder1
        du:
        Encoder_Msg_Data[0] = 0x2B;
        Encoder_Msg_Data[1] = 0x04;//2004对象字典
        Encoder_Msg_Data[2] = 0x20;
        Encoder_Msg_Data[3] = 0x00;
        Encoder_Msg_Data[4] = 0x01;//编码器清零标志位为1
        Encoder_Msg_Data[5] = 0x00;
        exit:Encoder_Msg_Data[4] = 0x00;//编码器清零标志位为0
      (default) -> Encoder1
    (default) -> Motor_Enable
    Second -> Goto
    Origin_Aciton_Move -> Wait [order 1] : [abs(Origin_Back_Angle)<=2]
    Wait -> Origin_Aciton_Move [order 1] : [abs(Origin_Back_Angle) > 2]
    Wait -> Motor_Stanby [order 2] : [after(1,sec)]
    Encoder1 -> Motor_Move : [ASSI_State==uint8(3)]
  (default) -> Init
  Init -> Pre_Operation_Mode
  Pre_Operation_Mode -> Move : [Str_Status]
  data: NMT_nodeorder output uint8; NMT_nodectrl output uint8; Enable_Operation_Ctrl output uint8; Quick_Stop_Ctrl output uint8; Enable_Voltage_Ctrl output uint8; Halt_Ctrl output uint8; Switch_On_Ctrl output uint8; Abs_or_Rel_Ctrl output uint8; New_Set_Point_Ctrl output uint8; Position_set output single; Encoder_Msg_Data output uint8 size=6; Original_Flag output double; Origin_Back_Angle input single; Steer_Go_Angle input int8; ASSI_State input uint8; Str_Status input uint8; Fault_Resrt output double; flag output double; enflag output double
  events: TmtNMTCAN output FUNCTION_CALL_EVENT; TmtRPDO1CAN output FUNCTION_CALL_EVENT; TmtSDOCAN output FUNCTION_CALL_EVENT
